simulink model "sampleModel1456"  (R2023a)
settings: Solver=VariableStepAuto  StartTime=0.0  StopTime=10.0  RelTol=1e-3
libraries: simulink x2, hdlsllib x2
settings Model: Creator=user1  LastModifiedBy=user1

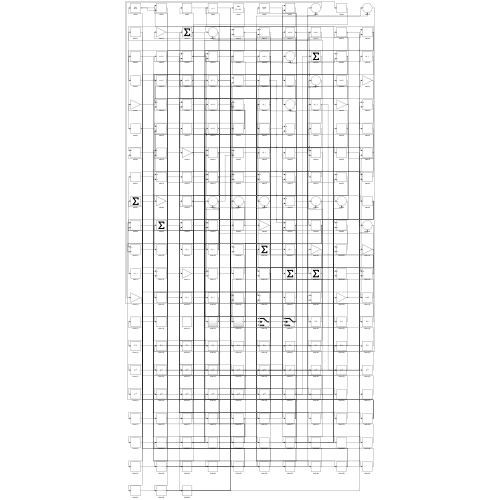
[thumbnail: Simulink's stored preview of the top-level diagram]
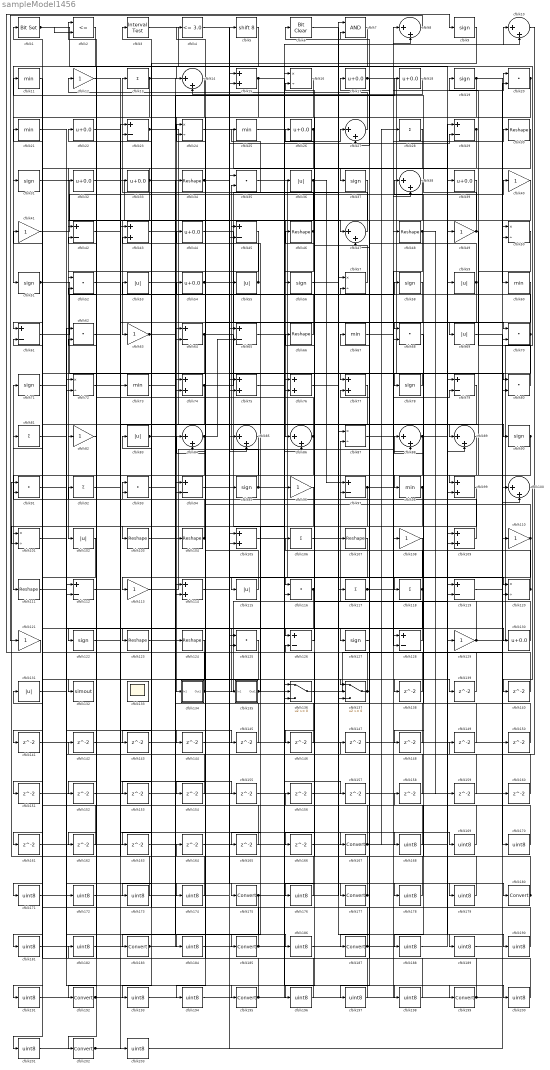
== system sampleModel1456 ==
  cfblk1 : simulink/Logic and Bit Operations/Bit Set  iBit=0
      settings: LibrarySourceBlock=|
      | hdlsllib/Logic and Bit
      | Operations/Bit Set
  cfblk{8,10,14,27,38,47,84..86,88..89,100} (12 alike) : Sum  Inputs=|++
  cfblk{16,24,50,57,72,87,101,120} (8 alike) : Product  Inputs=*/  RndMeth=Zero  SaturateOnIntegerOverflow=on
  cfblk{36,53,55,59,69,83,102,115,131} (9 alike) : Abs  SaturateOnIntegerOverflow=off
  cfblk{30,34,46,48,66,103..104,107,111,123..124} (11 alike) : Reshape
  cfblk{15,43,74..77,99,105,109,114} (10 alike) : Sum
  cfblk{13,28,81,92,106,117..118} (7 alike) : Sum  Inputs=+
  cfblk{12,40..41,49,63,82,96,108,110,113,121,129} (12 alike) : Gain
  cfblk{11,21,25,60,67,73,98} (7 alike) : MinMax
  cfblk{23,29,42,45,61,64..65,79,94,97,112,119,126,128} (14 alike) : Sum  Inputs=+-
  cfblk{20,35,52,62,68,70,80,91,93,116,125} (11 alike) : DotProduct  OutDataTypeStr=Inherit: Inherit via internal rule
  cfblk{9,19,31,37,51,56,58,71,78,90,95,122,127} (13 alike) : Signum
  cfblk{17..18,22,26,32..33,39,44,54,130} (10 alike) : Bias  Bias=0.0  SaturateOnIntegerOverflow=off
  cfblk132 : ToWorkspace  VariableName=simout  SaveFormat=Timeseries  SampleTime=-1
  cfblk133 : Scope
      settings: Floating=on
  cfblk134 : Subsystem
      settings: LibrarySourceBlock=|
      | hdlsllib/Ports &
      | Subsystems/Subsystem
  cfblk135 : Subsystem
      settings: LibrarySourceBlock=|
      | hdlsllib/Ports &
      | Subsystems/Subsystem
  cfblk136 : Switch  SaturateOnIntegerOverflow=off  InputSameDT=off
  cfblk137 : Switch  SaturateOnIntegerOverflow=off  InputSameDT=off
  cfblk{138..166} (29 alike) : Delay  SampleTime=1
  cfblk{167,175,177,180,183,185,187,192,195,199,202} (11 alike) : DataTypeConversion  SaturateOnIntegerOverflow=off  RndMeth=Floor
  cfblk{168..174,176,178..179,181..182,184,186,188..191,193..194,196..198,200..201,203} (26 alike) : DataTypeConversion  OutDataTypeStr=uint8  SaturateOnIntegerOverflow=off  RndMeth=Floor
  cfblk2 : RelationalOperator  Operator=<=  OutDataTypeStr=boolean  InputSameDT=off
  cfblk3 : hdlsllib/Logic and Bit Operations/Interval Test  IntervalClosedRight=on  uplimit=0.5  IntervalClosedLeft=on  lowlimit=-0.5  OutDataTypeStr=boolean
  cfblk4 : hdlsllib/Logic and Bit Operations/Compare To Constant  relop=<=  const=3.0  OutDataTypeStr=boolean
  cfblk5 : ArithShift  BitShiftNumber=8
  cfblk6 : simulink/Logic and Bit Operations/Bit Clear  iBit=0
      settings: LibrarySourceBlock=|
      | hdlsllib/Logic and Bit
      | Operations/Bit Clear
  cfblk7 : Logic  AllPortsSameDT=off  OutDataTypeStr=boolean
  wires:
  cfblk14/1 -> cfblk134/1(In1)
  cfblk36/1 -> cfblk63/1, cfblk97/1
  cfblk97/1 -> cfblk115/1, cfblk79/2
  cfblk70/1 -> cfblk53/1, cfblk125/2
  cfblk75/1 -> cfblk199/1
  cfblk129/1 -> cfblk14/1, cfblk77/2
  cfblk35/1 -> cfblk120/1
  cfblk13/1 -> cfblk51/1, cfblk168/1
  cfblk9/1 -> cfblk22/1
  cfblk96/1 -> cfblk183/1
  cfblk92/1 -> cfblk175/1
  cfblk46/1 -> cfblk13/1, cfblk56/1
  cfblk28/1 -> cfblk37/1
  cfblk98/1 -> cfblk101/2, cfblk165/1, cfblk191/1
  cfblk24/1 -> cfblk119/1
  cfblk137/1 -> cfblk17/1, cfblk24/2
  cfblk26/1 -> cfblk102/1, cfblk72/2
  cfblk117/1 -> cfblk8/1, cfblk67/1
  cfblk5/1 -> cfblk202/1
  cfblk84/1 -> cfblk111/1, cfblk65/2
  cfblk40/1 -> cfblk86/1
  cfblk44/1 -> cfblk69/1
  cfblk8/1 -> cfblk121/1
  cfblk109/1 -> cfblk93/1
  cfblk31/1 -> cfblk47/1
  cfblk105/1 -> cfblk36/1
  cfblk121/1 -> cfblk9/1
  cfblk95/1 -> cfblk35/2, cfblk27/1
  cfblk104/1 -> cfblk71/1, cfblk62/2
  cfblk23/1 -> cfblk88/2, cfblk18/1
  cfblk17/1 -> cfblk80/1, cfblk27/2
  cfblk45/1 -> cfblk122/1
  cfblk130/1 -> cfblk87/2
  cfblk15/1 -> cfblk52/1, cfblk200/1
  cfblk27/1 -> cfblk12/1
  cfblk43/1 -> cfblk177/1
  cfblk89/1 -> cfblk123/1
  cfblk128/1 -> cfblk66/1
  cfblk74/1 -> cfblk7/1, cfblk201/1
  cfblk6/1 -> cfblk117/1
  cfblk86/1 -> cfblk42/2, cfblk154/1
  cfblk4/1 -> cfblk167/1
  cfblk18/1 -> cfblk14/2
  cfblk113/1 -> cfblk20/1
  cfblk94/1 -> cfblk180/1
  cfblk68/1 -> cfblk118/1
  cfblk82/1 -> cfblk132/1
  cfblk110/1 -> cfblk116/1, cfblk84/2, cfblk166/1
  cfblk51/1 -> cfblk100/1, cfblk171/1
  cfblk2/1 -> cfblk31/1
  cfblk87/1 -> cfblk30/1
  cfblk19/1 -> cfblk60/1, cfblk126/1
  cfblk29/1 -> cfblk101/1, cfblk146/1
  cfblk72/1 -> cfblk73/1
  cfblk66/1 -> cfblk3/1
  cfblk83/1 -> cfblk127/1, cfblk57/2
  cfblk64/1 -> cfblk116/2, cfblk161/1
  cfblk54/1 -> cfblk104/1, cfblk29/2
  cfblk136/1 -> cfblk50/1
  cfblk38/1 -> cfblk82/1
  cfblk49/1 -> cfblk11/1, cfblk99/1
  cfblk34/1 -> cfblk119/2, cfblk78/1
  cfblk119/1 -> cfblk100/2
  cfblk57/1 -> cfblk16/2
  cfblk126/1 -> cfblk106/1
  cfblk120/1 -> cfblk38/1, cfblk26/1
  cfblk41/1 -> cfblk40/1
  cfblk116/1 -> cfblk176/1, cfblk181/1
  cfblk21/1 -> cfblk130/1
  cfblk55/1 -> cfblk23/2, cfblk44/1
  cfblk3/1 -> cfblk65/1
  cfblk59/1 -> cfblk128/2, cfblk6/1
  cfblk53/1 -> cfblk74/2
  cfblk56/1 -> cfblk10/1
  cfblk93/1 -> cfblk58/1
  cfblk115/1 -> cfblk24/1
  cfblk58/1 -> cfblk124/1
  cfblk67/1 -> cfblk38/2
  cfblk81/1 -> cfblk195/1
  cfblk85/1 -> cfblk192/1
  cfblk118/1 -> cfblk46/1, cfblk135/1(In1)
  cfblk106/1 -> cfblk107/1
  cfblk30/1 -> cfblk136/2
  cfblk78/1 -> cfblk77/1
  cfblk52/1 -> cfblk70/1
  cfblk79/1 -> cfblk113/1
  cfblk20/1 -> cfblk114/2, cfblk194/1
  cfblk114/1 -> cfblk95/1
  cfblk32/1 -> cfblk86/2
  cfblk65/1 -> cfblk68/1
  cfblk48/1 -> cfblk68/2, cfblk159/1
  cfblk33/1 -> cfblk32/1, cfblk45/2, cfblk42/1
  cfblk63/1 -> cfblk138/1, cfblk139/1
  cfblk108/1 -> cfblk185/1
  cfblk103/1 -> cfblk34/1
  cfblk88/1 -> cfblk190/1, cfblk196/1
  cfblk39/1 -> cfblk187/1
  cfblk47/1 -> cfblk25/1
  cfblk50/1 -> cfblk89/1
  cfblk60/1 -> cfblk105/2
  cfblk80/1 -> cfblk19/1
  cfblk134/1(Out1) -> cfblk2/1, cfblk29/1
  cfblk11/1 -> cfblk61/1
  cfblk61/1 -> cfblk15/2
  cfblk90/1 -> cfblk98/1, cfblk103/1, cfblk109/2, cfblk188/1
  cfblk1/1 -> cfblk49/1, cfblk2/2
  cfblk12/1 -> cfblk90/1
  cfblk123/1 -> cfblk137/1
  cfblk127/1 -> cfblk47/2
  cfblk135/1(Out1) -> cfblk45/1, cfblk10/2
  cfblk138/1 -> cfblk15/1
  cfblk139/1 -> cfblk61/2
  cfblk100/1 -> cfblk140/1
  cfblk140/1 -> cfblk7/2
  cfblk102/1 -> cfblk141/1
  cfblk141/1 -> cfblk114/1
  cfblk37/1 -> cfblk143/1
  cfblk143/1 -> cfblk70/2
  cfblk71/1 -> cfblk144/1
  cfblk144/1 -> cfblk120/2
  cfblk62/1 -> cfblk145/1
  cfblk145/1 -> cfblk105/1
  cfblk146/1 -> cfblk136/1
  cfblk99/1 -> cfblk148/1
  cfblk148/1 -> cfblk35/1
  cfblk10/1 -> cfblk149/1
  cfblk149/1 -> cfblk74/1
  cfblk150/1 -> cfblk88/1
  cfblk125/1 -> cfblk151/1
  cfblk151/1 -> cfblk137/2
  cfblk16/1 -> cfblk152/1
  cfblk152/1 -> cfblk8/2
  cfblk107/1 -> cfblk153/1
  cfblk153/1 -> cfblk20/2
  cfblk154/1 -> cfblk72/1
  cfblk42/1 -> cfblk155/1
  cfblk155/1 -> cfblk87/1
  cfblk156/1 -> cfblk50/2
  cfblk25/1 -> cfblk157/1
  cfblk157/1 -> cfblk80/2
  cfblk158/1 -> cfblk97/2
  cfblk159/1 -> cfblk64/1
  cfblk160/1 -> cfblk79/1
  cfblk161/1 -> cfblk136/3
  cfblk77/1 -> cfblk162/1
  cfblk162/1 -> cfblk1/1
  cfblk124/1 -> cfblk163/1
  cfblk163/1 -> cfblk93/2
  cfblk164/1 -> cfblk137/3
  cfblk165/1 -> cfblk23/1
  cfblk166/1 -> cfblk89/2
  cfblk167/1 -> cfblk99/2, cfblk54/1, cfblk28/1
  cfblk168/1 -> cfblk4/1
  cfblk112/1 -> cfblk169/1
  cfblk169/1 -> cfblk142/1
  cfblk69/1 -> cfblk170/1
  cfblk170/1 -> cfblk112/1
  cfblk171/1 -> cfblk112/2
  cfblk91/1 -> cfblk172/1
  cfblk172/1 -> cfblk55/1
  cfblk7/1 -> cfblk173/1
  cfblk173/1 -> cfblk91/1
  cfblk142/1 -> cfblk174/1
  cfblk174/1 -> cfblk91/2
  cfblk175/1 -> cfblk57/1, cfblk193/1
  cfblk176/1 -> cfblk92/1
  cfblk177/1 -> cfblk41/1, cfblk126/2, cfblk16/1
  cfblk22/1 -> cfblk178/1
  cfblk178/1 -> cfblk43/1
  cfblk111/1 -> cfblk179/1
  cfblk179/1 -> cfblk43/2
  cfblk180/1 -> cfblk158/1, cfblk156/1, cfblk83/1, cfblk128/1
  cfblk181/1 -> cfblk94/1
  cfblk182/1 -> cfblk94/2
  cfblk183/1 -> cfblk64/2, cfblk59/1
  cfblk131/1 -> cfblk184/1
  cfblk184/1 -> cfblk96/1
  cfblk185/1 -> cfblk33/1, cfblk131/1
  cfblk73/1 -> cfblk186/1
  cfblk186/1 -> cfblk108/1
  cfblk187/1 -> cfblk164/1, cfblk109/1, cfblk129/1
  cfblk188/1 -> cfblk39/1
  cfblk76/1 -> cfblk189/1
  cfblk189/1 -> cfblk110/1
  cfblk190/1 -> cfblk76/1
  cfblk191/1 -> cfblk76/2
  cfblk192/1 -> cfblk160/1, cfblk48/1
  cfblk193/1 -> cfblk85/1
  cfblk194/1 -> cfblk85/2
  cfblk195/1 -> cfblk62/1, cfblk21/1
  cfblk196/1 -> cfblk81/1
  cfblk147/1 -> cfblk197/1
  cfblk197/1 -> cfblk52/2
  cfblk101/1 -> cfblk198/1
  cfblk198/1 -> cfblk147/1
  cfblk199/1 -> cfblk182/1, cfblk84/1
  cfblk200/1 -> cfblk75/1
  cfblk201/1 -> cfblk75/2
  cfblk202/1 -> cfblk150/1, cfblk125/1
  cfblk122/1 -> cfblk203/1
  cfblk203/1 -> cfblk5/1

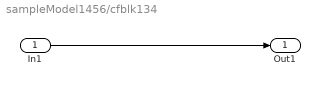
== system sampleModel1456/cfblk134 ==
  In1 : Inport
  Out1 : Outport
  wires:
  In1/1 -> Out1/1

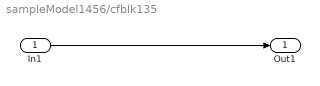
== system sampleModel1456/cfblk135 ==
  In1 : Inport
  Out1 : Outport
  wires:
  In1/1 -> Out1/1
